simulink model "lab04"  (Simulink 10.3)
settings: Solver=FixedStepAuto  StartTime=0.0  StopTime=100  FixedStep=0.001768  RelTol=1e-3
values from neighbouring files (symbols this model uses):
  k_d = 0.00416035381008    [lab03.mat]    (also in lab04.mat = 0.00114359359927; lab05.mat = 0.00883154670201; lab06.mat = 0.05; lab07.mat = 0.00883154670201)
  k_i = 0    [lab04.mat]    (also in lab05.mat; lab06.mat; lab07.mat)
  k_p = 2    [lab02.mat]    (also in lab03.mat = 0.256097247605; lab04.mat = 0.137612608424; lab05.mat = 0.280842058008; lab06.mat = 0.012)
undefined symbols (not defined in the file or in its folder): G_p
libraries: simulink x1
settings Model: Creator=kisdev  LastModifiedBy=kisdev
settings SolverCC: AlgebraicLoopSolver=Auto
settings DataIOCC: SaveFormat=Dataset  SignalLoggingSaveFormat=Dataset  ReturnWorkspaceOutputs=on
settings OptimizationCC: ExpressionDepthLimit=128  LifeSpan=auto
settings DebuggingCC: UnderspecifiedInitializationDetection=Simplified  MergeDetectMultiDrivingBlocksExec=error  FcnCallInpInsideContextMsg=error  StateNameClashWarn=none  SFUnexpectedBacktrackingDiag=error  SFNoUnconditionalDefaultTransitionDiag=error  SFExecutionAtInitializationDiag=warning  SFMachineParentedDataDiag=error  ArithmeticOperatorsInVariantConditions=error
settings HardwareCC: ProdBitPerPointer=64  ProdBitPerSizeT=64  ProdBitPerPtrDiffT=64  ProdLargestAtomicFloat=Float  ProdIntDivRoundTo=Zero  ProdEndianess=LittleEndian  ProdWordSize=64  ProdHWDeviceType=Intel->x86-64 (Windows64)
settings ModelReferenceCC: PropagateSignalLabelsOutOfModel=on
settings SFSimCC: SimUseLocalCustomCode=on  CustomCodeUndefinedFunction=FilterOut
settings RTWCC: RTWUseLocalCustomCode=on
settings CodeAppCC: StateflowObjectComments=off
settings GRTTargetCC: TargetLangStandard=C99 (ISO)  CombineOutputUpdateFcns=on  GRTInterface=off
settings ConfigComp: CovMetricSettings=dwe  CovSaveCumulativeToWorkspaceVar=off  CovSaveSingleToWorkspaceVar=off  CovExternalEMLEnable=on

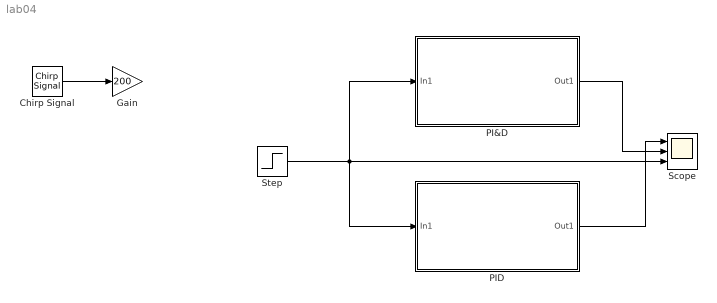
== system lab04 ==
  Chirp Signal : simulink/Sources/Chirp Signal  f1=0.1  T=100  f2=10
  Gain : Gain  Gain=200
  PI&D : Subsystem
  PID : Subsystem
  Scope : Scope  NumInputPorts=3
  Step : Step  Time=0  After=200  SampleTime=0
  wires:
  PI&D/1(Out1) -> Scope/2
  Chirp Signal/1 -> Gain/1
  PID/1(Out1) -> Scope/1
  Step/1 -> PI&D/1(In1), PID/1(In1), Scope/3

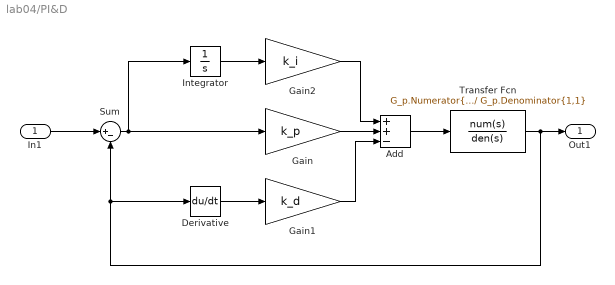
== system lab04/PI&D ==
  In1 : Inport
  Add : Sum  Inputs=++-
  Derivative : Derivative
  Gain : Gain  Gain=k_p
  Gain1 : Gain  Gain=k_d
  Gain2 : Gain  Gain=k_i
  Integrator : Integrator
  Sum : Sum  Inputs=|+-
  Transfer Fcn : TransferFcn  Numerator=G_p.Numerator{1,1}  Denominator=G_p.Denominator{1,1}
  Out1 : Outport
  wires:
  Transfer Fcn/1 -> Sum/2, Derivative/1, Out1/1
  Gain/1 -> Add/2
  Gain1/1 -> Add/3
  Derivative/1 -> Gain1/1
  In1/1 -> Sum/1
  Sum/1 -> Gain/1, Integrator/1
  Add/1 -> Transfer Fcn/1
  Integrator/1 -> Gain2/1
  Gain2/1 -> Add/1

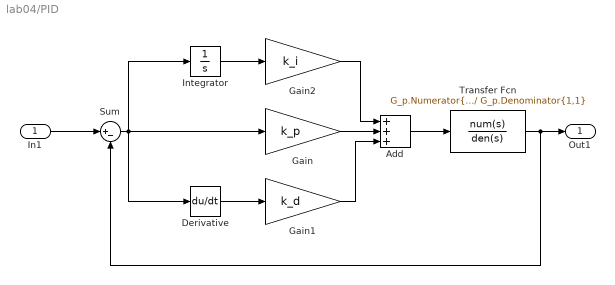
== system lab04/PID ==
  In1 : Inport
  Add : Sum  Inputs=+++
  Derivative : Derivative
  Gain : Gain  Gain=k_p
  Gain1 : Gain  Gain=k_d
  Gain2 : Gain  Gain=k_i
  Integrator : Integrator
  Sum : Sum  Inputs=|+-
  Transfer Fcn : TransferFcn  Numerator=G_p.Numerator{1,1}  Denominator=G_p.Denominator{1,1}
  Out1 : Outport
  wires:
  Transfer Fcn/1 -> Sum/2, Out1/1
  Gain/1 -> Add/2
  Gain1/1 -> Add/3
  Derivative/1 -> Gain1/1
  In1/1 -> Sum/1
  Sum/1 -> Derivative/1, Gain/1, Integrator/1
  Add/1 -> Transfer Fcn/1
  Integrator/1 -> Gain2/1
  Gain2/1 -> Add/1
